simulink model "TrackingComparison"  (R2018a)
settings: Solver=VariableStepAuto  StartTime=0.0  StopTime=10.0  RelTol=1e-3
PreLoadFcn:
  | modelDir = fileparts(get_param(bdroot, 'FileName'));
  | addpath(fullfile(modelDir,'../../Misc'));
settings Model: Creator=Thomas  LastModifiedBy=Thomas

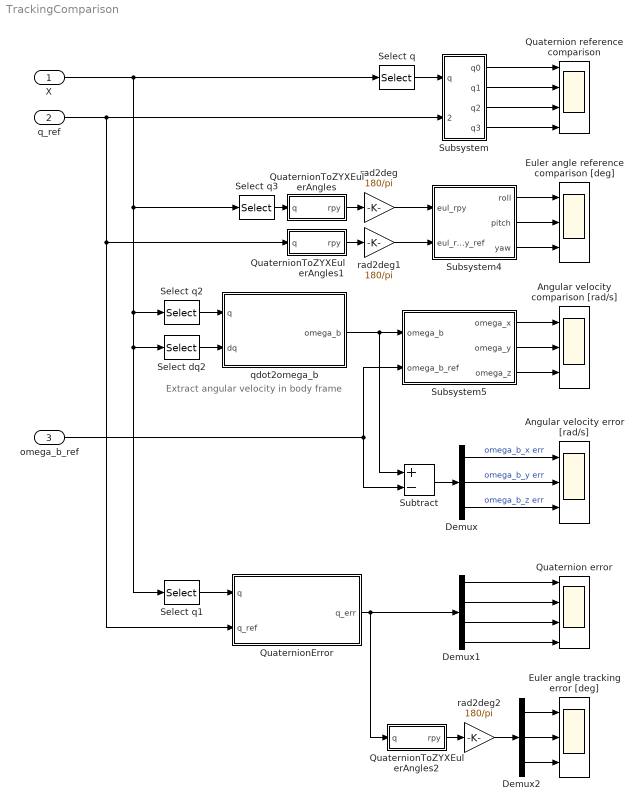
== system TrackingComparison ==
  note: Extract angular velocity in body frame
  X : Inport
  q_ref : Inport  Port=2
  omega_b_ref : Inport  Port=3
  Angular velocity comparison [rad/s] : Scope  NumInputPorts=3
  Angular velocity error [rad/s] : Scope  NumInputPorts=3
  Demux : Demux  Outputs=3
  Demux1 : Demux
  Demux2 : Demux  Outputs=3
  Euler angle reference comparison [deg] : Scope  NumInputPorts=3
  Euler angle tracking error [deg] : Scope  NumInputPorts=3
  Quaternion error : Scope  NumInputPorts=4
  Quaternion reference comparison : Scope  NumInputPorts=4
  QuaternionError : MATLAB Function  TreatAsAtomicUnit=on
  QuaternionToZYXEulerAngles : MATLAB Function  TreatAsAtomicUnit=on
  QuaternionToZYXEulerAngles1 : MATLAB Function  TreatAsAtomicUnit=on
  QuaternionToZYXEulerAngles2 : MATLAB Function  TreatAsAtomicUnit=on
  Select dq2 : Selector  InputPortWidth=12  IndexOptions=Index vector (dialog)  Indices=[9,10,11,12]  OutputSizes=1
  Select q{,1..3} (4 alike) : Selector  InputPortWidth=12  IndexOptions=Index vector (dialog)  Indices=[3,4,5,6]  OutputSizes=1
  Subsystem : Subsystem
  Subsystem4 : Subsystem
  Subsystem5 : Subsystem
  Subtract : Sum  Inputs=+-
  qdot2omega_b : MATLAB Function  TreatAsAtomicUnit=on
  rad2deg : Gain  Gain=180/pi
  rad2deg1 : Gain  Gain=180/pi
  rad2deg2 : Gain  Gain=180/pi
  wires:
  Subsystem/1(q0) -> Quaternion reference comparison/1
  Subsystem/4(q3) -> Quaternion reference comparison/4
  Subsystem/3(q2) -> Quaternion reference comparison/3
  Subsystem/2(q1) -> Quaternion reference comparison/2
  Select q/1 -> Subsystem/1(q)
  q_ref/1 -> Subsystem/2(q_ref), QuaternionError/2(q_ref), QuaternionToZYXEulerAngles1/1(q)
  X/1 -> Select q/1, Select q3/1, Select q2/1, Select q1/1, Select dq2/1
  Subsystem4/2(pitch) -> Euler angle reference comparison [deg]/2
  Subsystem4/1(roll) -> Euler angle reference comparison [deg]/1
  rad2deg/1 -> Subsystem4/1(eul_rpy)
  Select q3/1 -> QuaternionToZYXEulerAngles/1(q)
  QuaternionToZYXEulerAngles/1(rpy) -> rad2deg/1
  rad2deg1/1 -> Subsystem4/2(eul_rpy_ref)
  Subsystem4/3(yaw) -> Euler angle reference comparison [deg]/3
  Subsystem5/1(omega_x) -> Angular velocity comparison [rad/s]/1
  qdot2omega_b/1(omega_b) -> Subtract/1, Subsystem5/1(omega_b)
  Select q2/1 -> qdot2omega_b/1(q)
  Select dq2/1 -> qdot2omega_b/2(dq)
  Subsystem5/2(omega_y) -> Angular velocity comparison [rad/s]/2
  omega_b_ref/1 -> Subtract/2, Subsystem5/2(omega_b_ref)
  Subsystem5/3(omega_z) -> Angular velocity comparison [rad/s]/3
  Demux/1 -> Angular velocity error [rad/s]/1  "omega_b_x err"
  Demux/2 -> Angular velocity error [rad/s]/2  "omega_b_y err"
  Demux/3 -> Angular velocity error [rad/s]/3  "omega_b_z err"
  Subtract/1 -> Demux/1
  Demux1/1 -> Quaternion error/1
  Demux1/2 -> Quaternion error/2
  Demux1/3 -> Quaternion error/3
  Demux1/4 -> Quaternion error/4
  QuaternionError/1(q_err) -> Demux1/1, QuaternionToZYXEulerAngles2/1(q)
  Select q1/1 -> QuaternionError/1(q)
  QuaternionToZYXEulerAngles2/1(rpy) -> rad2deg2/1
  Demux2/3 -> Euler angle tracking error [deg]/3
  Demux2/2 -> Euler angle tracking error [deg]/2
  Demux2/1 -> Euler angle tracking error [deg]/1
  rad2deg2/1 -> Demux2/1
  QuaternionToZYXEulerAngles1/1(rpy) -> rad2deg1/1

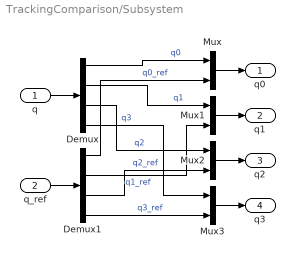
== system TrackingComparison/Subsystem ==
  q : Inport
  q_ref : Inport  Port=2
  Demux : Demux
  Demux1 : Demux
  Mux{,1..3} (4 alike) : Mux  Inputs=2
  q0 : Outport
  q1 : Outport  Port=2
  q2 : Outport  Port=3
  q3 : Outport  Port=4
  wires:
  Demux1/2 -> Mux1/2  "q1_ref"
  Demux1/3 -> Mux2/2  "q2_ref"
  Demux/4 -> Mux3/1  "q3"
  Mux1/1 -> q1/1
  Demux1/4 -> Mux3/2  "q3_ref"
  Demux/3 -> Mux2/1  "q2"
  Demux1/1 -> Mux/2  "q0_ref"
  Mux2/1 -> q2/1
  q_ref/1 -> Demux1/1
  Demux/1 -> Mux/1  "q0"
  Mux/1 -> q0/1
  Demux/2 -> Mux1/1  "q1"
  q/1 -> Demux/1
  Mux3/1 -> q3/1

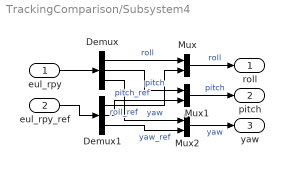
== system TrackingComparison/Subsystem4 ==
  eul_rpy : Inport
  eul_rpy_ref : Inport  Port=2
  Demux : Demux  Outputs=3
  Demux1 : Demux  Outputs=3
  Mux : Mux  Inputs=2
  Mux1 : Mux  Inputs=2
  Mux2 : Mux  Inputs=2
  roll : Outport
  pitch : Outport  Port=2
  yaw : Outport  Port=3
  wires:
  Demux/2 -> Mux1/1  "pitch"
  Demux/1 -> Mux/1  "roll"
  Mux/1 -> roll/1  "roll"
  Demux/3 -> Mux2/1  "yaw"
  Demux1/3 -> Mux2/2  "yaw_ref"
  eul_rpy/1 -> Demux/1
  Demux1/1 -> Mux/2  "roll_ref"
  Demux1/2 -> Mux1/2  "pitch_ref"
  Mux2/1 -> yaw/1  "yaw"
  eul_rpy_ref/1 -> Demux1/1
  Mux1/1 -> pitch/1  "pitch"

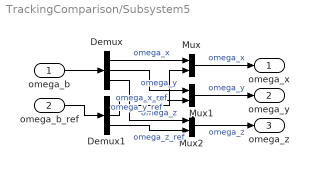
== system TrackingComparison/Subsystem5 ==
  omega_b : Inport
  omega_b_ref : Inport  Port=2
  Demux : Demux  Outputs=3
  Demux1 : Demux  Outputs=3
  Mux : Mux  Inputs=2
  Mux1 : Mux  Inputs=2
  Mux2 : Mux  Inputs=2
  omega_x : Outport
  omega_y : Outport  Port=2
  omega_z : Outport  Port=3
  wires:
  Demux/2 -> Mux1/1  "omega_y"
  Demux/1 -> Mux/1  "omega_x"
  Mux/1 -> omega_x/1  "omega_x"
  Demux/3 -> Mux2/1  "omega_z"
  Demux1/3 -> Mux2/2  "omega_z_ref"
  omega_b/1 -> Demux/1
  Demux1/1 -> Mux/2  "omega_x_ref"
  Demux1/2 -> Mux1/2  "omega_y_ref"
  Mux2/1 -> omega_z/1  "omega_z"
  omega_b_ref/1 -> Demux1/1
  Mux1/1 -> omega_y/1  "omega_y"

== matlab function TrackingComparison/QuaternionToZYXEulerAngles ==
  data: q input; rpy output
function rpy = Quaternion2ZYXEulerAngles(q)
    rpy = Quaternion2ZYXEulerAngles(q);
end

== matlab function TrackingComparison/QuaternionToZYXEulerAngles1 ==
  data: q input; rpy output
function rpy = Quaternion2ZYXEulerAngles(q)
    rpy = Quaternion2ZYXEulerAngles(q);
end

== matlab function TrackingComparison/qdot2omega_b ==
  data: q input; omega_b output; dq input
function omega_b = qdot2omega_b(q, dq)
    omega_b = qdot2omega_b(q, dq);
end

== matlab function TrackingComparison/QuaternionError ==
  data: q input; q_err output; q_ref input
function q_err = QuaternionError(q, q_ref)
    q_err = QuaternionError(q, q_ref);
end

== matlab function TrackingComparison/QuaternionToZYXEulerAngles2 ==
  data: q input; rpy output
function rpy = Quaternion2ZYXEulerAngles(q)
    rpy = Quaternion2ZYXEulerAngles(q);
end
